simulink model "CLIK_2nd_order"  (R2023b)
settings: Solver=ode1  StartTime=0.0  StopTime=50  FixedStep=Tc  RelTol=1e-3
values from neighbouring files (symbols this model uses):
  Tc = 0.001    [scara_parameters.m]
undefined symbols (not defined in the file or in its folder): DiscIntNeverNeededParam, K_D, K_P, q0
settings Model: Creator=emman  LastModifiedBy=emman

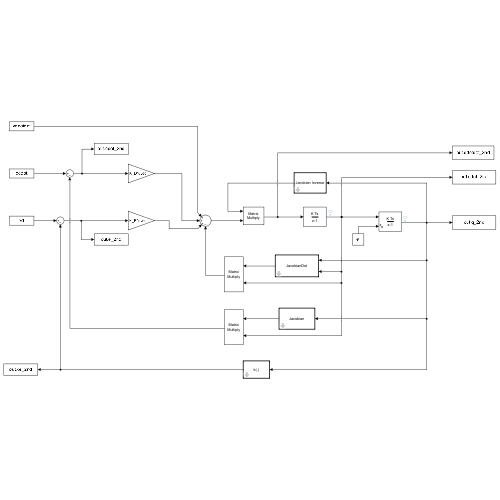
[thumbnail: Simulink's stored preview of the top-level diagram]
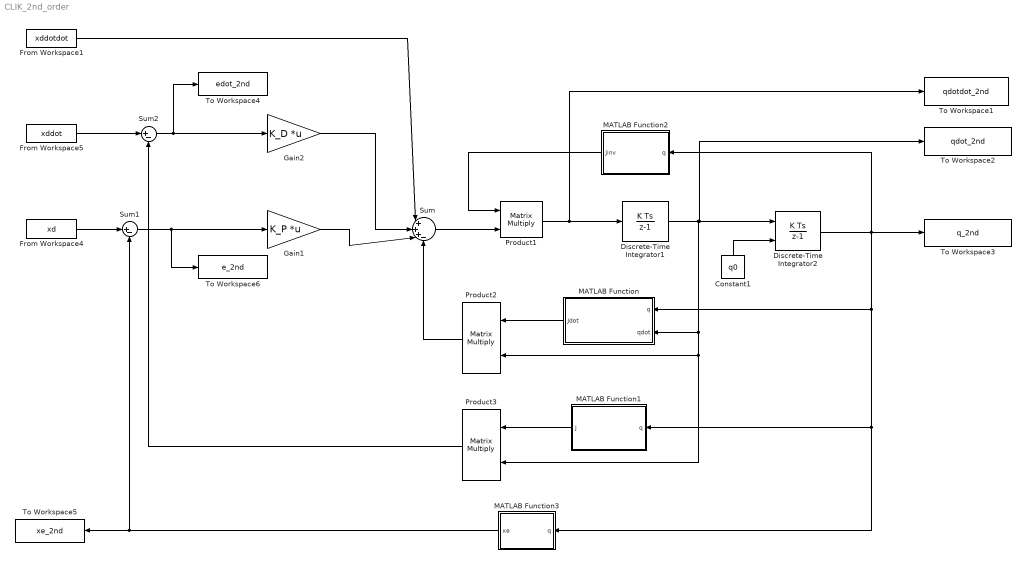
== system CLIK_2nd_order ==
  Constant1 : Constant  Value=q0
  Discrete-Time Integrator1 : DiscreteIntegrator  InitialCondition=[0 0 0 0]'  SampleTime=Tc  ICPrevOutput=DiscIntNeverNeededParam  ICPrevScaledInput=DiscIntNeverNeededParam
  Discrete-Time Integrator2 : DiscreteIntegrator  InitialConditionSource=external  InitialCondition=q0  SampleTime=Tc  ICPrevOutput=DiscIntNeverNeededParam  ICPrevScaledInput=DiscIntNeverNeededParam
  From Workspace1 : FromWorkspace  VariableName=xddotdot  SampleTime=Tc
  From Workspace4 : FromWorkspace  VariableName=xd  SampleTime=Tc
  From Workspace5 : FromWorkspace  VariableName=xddot  SampleTime=Tc
  Gain1 : Gain  Gain=K_P  Multiplication=Matrix(K*u) (u vector)
  Gain2 : Gain  Gain=K_D  Multiplication=Matrix(K*u) (u vector)
  MATLAB Function : MATLAB Function  TreatAsAtomicUnit=on
  MATLAB Function1 : MATLAB Function  TreatAsAtomicUnit=on
  MATLAB Function2 : MATLAB Function  TreatAsAtomicUnit=on
  MATLAB Function3 : MATLAB Function  TreatAsAtomicUnit=on
  Product1 : Product  Multiplication=Matrix(*)
  Product2 : Product  Multiplication=Matrix(*)
  Product3 : Product  Multiplication=Matrix(*)
  Sum : Sum  Inputs=|+++-
  Sum1 : Sum  Inputs=|+-
  Sum2 : Sum  Inputs=|+-
  To Workspace1 : ToWorkspace  VariableName=qdotdot_2nd  SaveFormat=Structure With Time  SampleTime=-1
  To Workspace2 : ToWorkspace  VariableName=qdot_2nd  SaveFormat=Structure With Time  SampleTime=-1
  To Workspace3 : ToWorkspace  VariableName=q_2nd  SaveFormat=Structure With Time  SampleTime=-1
  To Workspace4 : ToWorkspace  VariableName=edot_2nd  SaveFormat=Structure With Time  SampleTime=-1
  To Workspace5 : ToWorkspace  VariableName=xe_2nd  SaveFormat=Structure With Time  SampleTime=-1
  To Workspace6 : ToWorkspace  VariableName=e_2nd  SaveFormat=Structure With Time  SampleTime=-1
  wires:
  From Workspace4/1 -> Sum1/1
  MATLAB Function3/1(xe) -> To Workspace5/1, Sum1/2
  MATLAB Function2/1(Jinv) -> Product1/1
  Gain1/1 -> Sum/3
  Sum/1 -> Product1/2
  Product1/1 -> Discrete-Time Integrator1/1, To Workspace1/1
  Sum1/1 -> To Workspace6/1, Gain1/1
  From Workspace5/1 -> Sum2/1
  Sum2/1 -> To Workspace4/1, Gain2/1
  Gain2/1 -> Sum/2
  From Workspace1/1 -> Sum/1
  Discrete-Time Integrator1/1 -> To Workspace2/1, Discrete-Time Integrator2/1, Product3/2, Product2/2, MATLAB Function/2(qdot)
  Constant1/1 -> Discrete-Time Integrator2/2
  Discrete-Time Integrator2/1 -> To Workspace3/1, MATLAB Function3/1(q), MATLAB Function1/1(q), MATLAB Function/1(q), MATLAB Function2/1(q)
  MATLAB Function/1(Jdot) -> Product2/1
  Product2/1 -> Sum/4
  MATLAB Function1/1(J) -> Product3/1
  Product3/1 -> Sum2/2

== matlab function CLIK_2nd_order/MATLAB Function ==
  data: q input; Jdot output; qdot input
function Jdot = JacobianDot(q,qdot)

    a1 = 0.5;
    a2 = 0.5;

    Jdot = [-a2*(qdot(1)+qdot(2))*cos(q(1)+q(2))-a1*qdot(1)*cos(q(1)) -a2*(qdot(1)+qdot(2))*cos(q(1)+q(2)) 0 0;
            -a2*(qdot(1)+qdot(2))*sin(q(1)+q(2))-a1*qdot(1)*sin(q(1)) -a2*(qdot(1)+qdot(2))*sin(q(1)+q(2)) 0 0;
            0 0 0 0;
            0 0 0 0];

end

== matlab function CLIK_2nd_order/MATLAB Function2 ==
  data: Jinv output; q input
function Jinv = JacobianInverse(q)

J = jacobian(q);

Jinv = inv(J);

end

== matlab function CLIK_2nd_order/MATLAB Function3 ==
  data: q input; xe output
function xe = DirKin(q)

    xe = k(q);

end

== matlab function CLIK_2nd_order/MATLAB Function1 ==
  data: q input; J output
function J = Jac(q)
    
    J = jacobian(q);

end
